simulink model "Drone_BBall_Developer"  (R2020a)
settings: Solver=FixedStepAuto  StartTime=0.0  StopTime=60  FixedStep=.001  RelTol=1e-3
values from neighbouring files (symbols this model uses):
  b = .25*m    (= 0.25)    [Run_Match.m]
  b_ball = .02*m_ball    (= 0.01)    [Run_Match.m]
  b_F_hook = 100    [Run_Match.m]
  b_F_hoop = m_ball * 50    (= 25)    [Run_Match.m]
  b_F_R = m * 20    (= 20)    [Run_Match.m]
  b_F_R_ball = m_ball * 10    (= 5)    [Run_Match.m]
  b_F_R_hook = m_hook * 100    (= 10)    [Run_Match.m]
  B_hook = r_hook^2*6*m_ball*g    (= 0.2943)    [Run_Match.m]
  b_hook = 0.05*m_hook    (= 0.005)    [Run_Match.m]
  b_tether = 1    [Run_Match.m]
  b_th = .1*J    (= 0.0192708333333)    [Run_Match.m]
  b_th_ball = .05*J_ball    (= 0.0009)    [Run_Match.m]
  b_x_net = 80*m_ball*g    (= 392.4)    [Run_Match.m]
  b_y_net = .4*m_ball*g    (= 1.962)    [Run_Match.m]
  drone = struct([])    [Run_Match.m]    (also in animate_drone_bball.m = [-r+w -r-w -r -r r r r+w r-w;             h    h  h  0 0 h  )
  g = 9.81    [Run_Match.m]
  J = 1/4*m*r^2 + 1/12*m*(2*(r+r_M_R))^2    (= 0.192708333333)    [Run_Match.m]
  J_ball = 2/5*m_ball*r_ball^2    (= 0.018)    [Run_Match.m]
  k_f = 4    [Run_Match.m]
  k_F_hook = 10000    [Run_Match.m]
  k_F_hoop = m_ball * 5000    (= 2500)    [Run_Match.m]
  k_F_R = m * 10000    (= 10000)    [Run_Match.m]
  k_F_R_ball = m_ball * 10000    (= 5000)    [Run_Match.m]
  k_F_R_hook = m_hook * 10000    (= 1000)    [Run_Match.m]
  k_tether = 40    [Run_Match.m]
  k_x_net = 200*m_ball*g    (= 981)    [Run_Match.m]
  k_y_net = .5*m_ball*g    (= 2.4525)    [Run_Match.m]
  L_tether = 1.0    (= 1)    [Run_Match.m]
  m = 1    [Run_Match.m]
  m_ball = .5    (= 0.5)    [Run_Match.m]
  m_hook = 0.1*m    (= 0.1)    [Run_Match.m]
  mu_f = .2    (= 0.2)    [Run_Match.m]
  mu_f_gnd = 0.5    [Run_Match.m]
  p_0 = [-5; 5]    [Run_Match.m]
  p_ball_0 = [0; r_ball]    [Run_Match.m]
  p_ball_dot_0 = [0; 12]    [Run_Match.m]
  p_emp = [0; -.4]    [Run_Match.m]
  p_emp_dot = [0; -5]    [Run_Match.m]
  p_hoop = [7.5 8; 8.5 8; -8.5 8; -7.5 8]'    [Run_Match.m]
  p_tether = [0; -0.259]    [Run_Match.m]
  r = 0.5    [Run_Match.m]    (also in animate_drone_bball.m = 0.475)
  r_ball = .3    (= 0.3)    [Run_Match.m]
  r_hook = 0.1    [Run_Match.m]
  r_M_R = 0.25*r    (= 0.125)    [Run_Match.m]
  T_0 = m*g    (= 9.81)    [Run_Match.m]
  T_max = 4*m*g    (= 39.24)    [Run_Match.m]
  T_tau = 0.1    [Run_Match.m]
undefined symbols (not defined in the file or in its folder): clock, M_max, sigbuilder_block, T_aux
libraries: dspswit3 x22, simulink x17, simulink_extras x3, dspmathops x2
(part 5 of 5)

== matlab function Drone_BBall_Developer/Drone 1 Controller/Predict Catch Position ==
  data: X_drone input; X_ball input; t_catch_prev input; X_catch output; t_catch output
function [X_catch,t_catch] = fcn(X_drone,X_ball,t_catch_prev)

% This function estimates how long it will take for the drone to catch the 
% ball, based on the current x-axis position and velocity of both the ball
% and the drone. It also estimates the state of the ball when the drone is
% expected to catch it. 
%
% This function assumes that the drone will accereate toward the ball at a
% constant rate. It takes into account a linear approximation of the drag 
% on the ball and drone using the Lambert W function (I had never heard of 
% it either!). I would not recommend changing the function.
%
% You can tune this function by setting the velocity operating points of 
% the drone and ball, and the horizontal aceleration of the drone, which
% are all used to make these estimates. If the estimate is good, the
% estimated catch time (plotted in the scope outside this function) should 
% be approximately constant as the drone moves to catch the ball.

% make sure these parameters match the main script
m = 1;
b = 0.25;
b_ball = 0.01;
m_ball = 0.5;
g = 9.81;
r_ball = 0.3;

% linearization operating point
v_lin_b = 3.125; % (m/s) [SET THIS] operating point velocity of ball (recoomended 3.125) 
v_lin_d = 1.75;  % (m/s) [SET THIS] operating point velocity of drone (recoomended 1.75)  

% internal variables
x_d_0 = X_drone(1);
x_d_dot_0 = X_drone(2);

x_b_0 = X_ball(1);
x_b_dot_0 = X_ball(2);
y_b_0 = X_ball(3);
y_b_dot_0 = X_ball(4);

% projectile motion parameters
a_d = 4.5; % (m/s^2) [SET THIS] magnitude of drone acceleration (recommended 4.5)
sign_ = sign(x_b_0 - x_d_0);

v_b = m_ball*g/(2*b_ball*v_lin_b);
v_d = m*a_d/(2*b*v_lin_d);

alpha = 0.85;

% can initialize t_catch_prev using projectile motion without drag
% t_raw = (delta_x_dot_0 + [1 -1]*sqrt(delta_x_dot_0^2 + 2*sign_*a_d*delta_x_0))/(sign_*a_d);
% t_catch = min(t_raw(t_raw>=0));

% or initialize based on previous value, which generally saves time
t_catch = t_catch_prev;

% conservative estimate of the minimum possible catch time
t_line = abs(x_b_0-x_d_0)/(max(sign_*x_d_dot_0,0)+max(-sign_*x_b_dot_0,0));
t_min = abs(x_b_0-x_d_0)/(a_d*t_line+max(0,sign_*x_d_dot_0)+max(0,-sign_*x_b_dot_0));

% check which branch of Lambert W function to use
A = 1 - sign_*x_d_dot_0/v_d;
B = 1 - sign_*(x_d_dot_0/v_d + a_d/v_d^2*(x_d_0 - x_b_0 - v_b*x_b_dot_0/g*(1-exp(-g*t_min/v_b))));
t_test = v_d/a_d * (lambert_w(-1, -A * exp(-B)) + B); % use approximation
if t_test < t_min
    branch = 0;
else
    branch = -1;
end

k_min = 1;
k_max = 10;

for k = k_min:k_max
    t_prev = real(t_catch);
    A = 1 - sign_*x_d_dot_0/v_d;
    B = 1 - sign_*(x_d_dot_0/v_d + a_d/v_d^2*(x_d_0 - x_b_0 - v_b*x_b_dot_0/g*(1-exp(-g*t_prev/v_b))));
    t_catch = v_d/a_d * (lambert_w(branch, -A * exp(-B)) + B); % use approximation
    t_catch = t_prev + .8^k*(t_catch-t_prev);
    if abs(t_catch - t_prev) < 0.001
        break
    else
%         t_catch = t_prev + .8^k*(t_catch-t_prev);
    end
end

max_bounce = 2;
t_n = [0 NaN(1,max_bounce)];
y_b_n = [y_b_0 NaN(1,max_bounce)];
y_b_dot_n = [y_b_dot_0 NaN(1,max_bounce)];

for bounce = 1:max_bounce
    E = m_ball*g*y_b_n(bounce) + 1/2*m_ball*y_b_dot_n(bounce)^2;
    y_bounce = min(y_b_n(bounce)-0.001,r_ball - 0.15*E/30);

    A = 1 + y_b_dot_n(bounce)/v_b;
    B = 1 + y_b_dot_n(bounce)/v_b + g/v_b^2*(y_b_n(bounce)-y_bounce);
    
    t_n_raw = v_b/g * (lambert_w([0 -1], -A * exp(-B)) + B); % use approximation
    if min(t_n_raw) >= 0
        t_n(bounce+1) = min(t_n_raw);
    else
        t_n(bounce+1) = max(t_n_raw);
    end
       
    y_b_n(bounce+1) = y_b_n(bounce) + v_b/g*(y_b_dot_n(bounce)+v_b)*(1-exp(-g*t_n(bounce+1)/v_b)) - v_b*t_n(bounce+1);
    y_b_dot_n(bounce+1) = -alpha * (y_b_dot_n(bounce)*exp(-g*t_n(bounce+1)/v_b) - v_b*(1-exp(-g*t_n(bounce+1)/v_b)));
end

X_catch = zeros(6,1);
X_catch(1) = x_b_0 + v_b/g*x_b_dot_0*(1-exp(-g*t_catch/v_b));
X_catch(2) = x_b_dot_0*exp(-g*t_catch/v_b);

bounce = max(1,sum(cumsum(t_n) <= t_catch));
X_catch(3) = y_b_n(bounce) + v_b/g*(y_b_dot_n(bounce)+v_b)*(1-exp(-g*(t_catch-t_n(bounce))/v_b)) - v_b*(t_catch-t_n(bounce));
X_catch(4) = y_b_dot_n(bounce)*exp(-g*(t_catch-t_n(bounce))/v_b) - v_b*(1-exp(-g*(t_catch-t_n(bounce))/v_b));
if X_catch(3) < r_ball
    X_catch(3:4) = [r_ball;0];
end

X_catch(5:6) = [0;0];

end

% helper function
function W = lambert_w(K,X)
% D. A. Barry, First version submitted to Mathworks on 23 June 2003
% Updated to remove warnings in the code, 31 March 2016
% andrew.barry@epfl.ch

% Various constants
em=-exp(-1); em9=-exp(-9); c13=1/3; em2=2/em; 
s2=sqrt(2); s21=2*s2-3; s22=4-3*s2; s23=s2-2;

W = zeros(size(K));

for n = 1:length(W)
    if K(n) == 0 % Calculations for crude Wp
        if X <= 20
            reta=s2*sqrt(max(0,1-X/em));
            an2=4.612634277343749*sqrt(sqrt(reta+1.09556884765625));
            W(n)=reta/(1+reta/(3+(s21*an2+s22)*reta/(s23*(an2+reta))))-1;
        else
            zl=log(X);
            W(n)=log(X/log(X/zl^exp(-1.124491989777808/(.4225028202459761+zl))));
        end
    else %  Calculations for crude Wm
        if X <= em9
            zl=log(max(0,-X));
            t=-1-zl;
            ts=sqrt(max(0,t));
            W(n)=zl-(2*ts)/(s2+(c13-t/(270+ts*127.0471381349219))*ts);
        else
            zl=log(max(0,-X));
            eta=2-em2*X;
            W(n)=log(X/log(-X/((1-.5043921323068457*(zl+1))*(sqrt(eta)+eta/3)+1)));
        end
    end
end

W = real(W);
end
